simulink model "fbw"  (R2020b)
settings: Solver=FixedStepAuto  StartTime=0.0  StopTime=10.0  FixedStep=0.02  RelTol=1e-3
undefined symbols (not defined in the file): DiscIntNeverNeededParam
libraries: simulink_extras x7, pid_lib x1
settings Model: Creator=Andreas  LastModifiedBy=Andreas

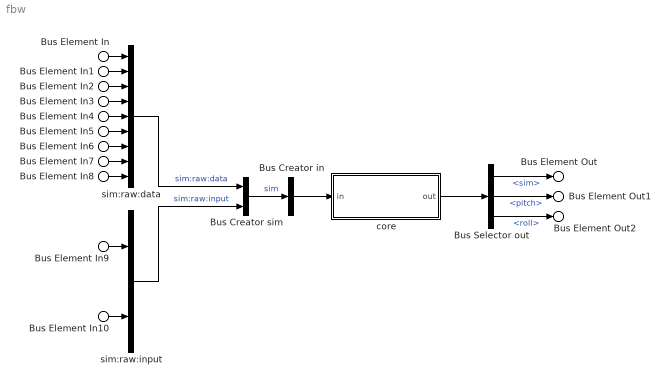
== system fbw ==
  Bus Element In : Inport  PortName=in  Element=sim.sim:raw:data.nz_g
  Bus Element In1 : Inport  PortName=in  Element=sim.sim:raw:data.Theta_deg
  Bus Element In2 : Inport  PortName=in  Element=sim.sim:raw:data.Phi_deg
  Bus Element In3 : Inport  PortName=in  Element=sim.sim:raw:data.qk_rad_s
  Bus Element In4 : Inport  PortName=in  Element=sim.sim:raw:data.rk_rad_s
  Bus Element In5 : Inport  PortName=in  Element=sim.sim:raw:data.pk_rad_s
  Bus Element In6 : Inport  PortName=in  Element=sim.sim:raw:data.Vk_kt
  Bus Element In7 : Inport  PortName=in  Element=sim.sim:raw:data.radio_height_ft
  Bus Element In8 : Inport  PortName=in  Element=sim.sim:raw:data.CG_percent_MAC
  Bus Element In9 : Inport  PortName=in  Element=sim.sim:raw:input.delta_eta_pos
  Bus Element In10 : Inport  PortName=in  Element=sim.sim:raw:input.delta_xi_pos
  Bus Creator sim : BusCreator  Inputs=2
  Bus Creator in : BusCreator  Inputs=1
  Bus Selector out : BusSelector  OutputSignals=sim,pitch,roll
  core : Subsystem
  sim:raw:data : BusCreator  Inputs=9
  sim:raw:input : BusCreator  Inputs=2
  Bus Element Out : Outport  PortName=out  Element=sim
  Bus Element Out1 : Outport  PortName=out  Element=pitch
  Bus Element Out2 : Outport  PortName=out  Element=roll
  wires:
  Bus Element In/1 -> sim:raw:data/1
  sim:raw:data/1 -> Bus Creator sim/1  "sim:raw:data"
  Bus Element In1/1 -> sim:raw:data/2
  Bus Element In2/1 -> sim:raw:data/3
  Bus Element In3/1 -> sim:raw:data/4
  Bus Element In4/1 -> sim:raw:data/5
  Bus Element In5/1 -> sim:raw:data/6
  Bus Element In6/1 -> sim:raw:data/7
  Bus Element In7/1 -> sim:raw:data/8
  Bus Element In8/1 -> sim:raw:data/9
  Bus Element In9/1 -> sim:raw:input/1
  Bus Element In10/1 -> sim:raw:input/2
  sim:raw:input/1 -> Bus Creator sim/2  "sim:raw:input"
  Bus Creator sim/1 -> Bus Creator in/1  "sim"
  Bus Creator in/1 -> core/1(in)
  core/1(out) -> Bus Selector out/1
  Bus Selector out/1 -> Bus Element Out/1  "<sim>"
  Bus Selector out/2 -> Bus Element Out1/1  "<pitch>"
  Bus Selector out/3 -> Bus Element Out2/1  "<roll>"

== system fbw/core ==
  in : Inport
  Data Computation : Subsystem
  Flight Laws : Subsystem
  Normalization : Subsystem
  Reverse Normalization : Subsystem
  out : Outport
  wires:
  Normalization/1(out) -> Data Computation/1(in)
  [B] -> Reverse Normalization/1(in)
  Data Computation/1(out) -> [A]
  [A] -> Flight Laws/1(in)
  Flight Laws/1(out) -> [B]
  Reverse Normalization/1(out) -> out/1
  in/1 -> Normalization/1(in)

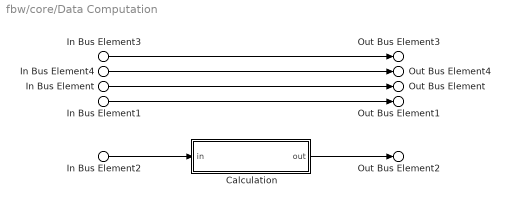
== system fbw/core/Data Computation ==
  In Bus Element2 : Inport  PortName=in
  In Bus Element : Inport  PortName=in  Element=sim.sim:data
  In Bus Element1 : Inport  PortName=in  Element=sim.sim:input
  In Bus Element3 : Inport  PortName=in  Element=sim.sim:raw:data
  In Bus Element4 : Inport  PortName=in  Element=sim.sim:raw:input
  Calculation : Subsystem
  Out Bus Element3 : Outport  PortName=out  Element=sim.sim:raw:data
  Out Bus Element4 : Outport  PortName=out  Element=sim.sim:raw:input
  Out Bus Element : Outport  PortName=out  Element=sim.sim:data
  Out Bus Element2 : Outport  PortName=out  Element=sim.sim:data:computed
  Out Bus Element1 : Outport  PortName=out  Element=sim.sim:input
  wires:
  In Bus Element4/1 -> Out Bus Element4/1
  In Bus Element3/1 -> Out Bus Element3/1
  Calculation/1(out) -> Out Bus Element2/1
  In Bus Element1/1 -> Out Bus Element1/1
  In Bus Element/1 -> Out Bus Element/1
  In Bus Element2/1 -> Calculation/1(in)

== system fbw/core/Flight Laws ==
  In Bus Element3 : Inport  PortName=in
  In Bus Element4 : Inport  PortName=in
  In Bus Element : Inport  PortName=in  Element=sim
  Bus Selector : BusSelector  OutputSignals=roll.roll:data:computed,roll.roll:normal,roll.roll:output  OutputAsBus=on
  Bus Selector1 : BusSelector  OutputSignals=pitch.pitch:data:computed,pitch.pitch:normal,pitch.pitch:protection:attitude:min,pitch.pitch:protection:attitude:max,pitch.pitch:vote,pitch.pitch:integrated,pitch.pitch:output  OutputAsBus=on
  Pitch : Subsystem
  Roll : Subsystem
  Out Bus Element : Outport  PortName=out  Element=sim
  Out Bus Element1 : Outport  PortName=out  Element=pitch
  Out Bus Element2 : Outport  PortName=out  Element=roll
  wires:
  Bus Selector1/1 -> Out Bus Element1/1
  Pitch/1(Output) -> Bus Selector1/1
  Bus Selector/1 -> Out Bus Element2/1
  Roll/1(out) -> Bus Selector/1
  In Bus Element4/1 -> Roll/1(in)
  In Bus Element/1 -> Out Bus Element/1
  In Bus Element3/1 -> Pitch/1(in)

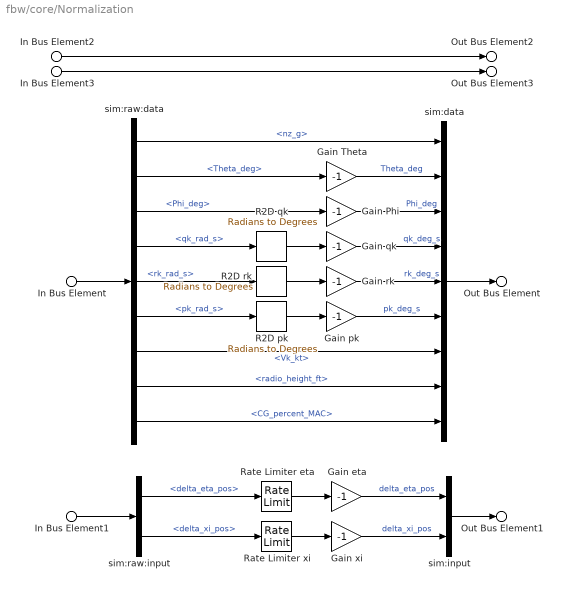
== system fbw/core/Normalization ==
  In Bus Element : Inport  PortName=in  Element=sim.sim:raw:data
  In Bus Element2 : Inport  PortName=in  Element=sim.sim:raw:data
  In Bus Element1 : Inport  PortName=in  Element=sim.sim:raw:input
  In Bus Element3 : Inport  PortName=in  Element=sim.sim:raw:input
  Gain Phi : Gain  Gain=-1
  Gain Theta : Gain  Gain=-1
  Gain eta : Gain  Gain=-1
  Gain pk : Gain  Gain=-1
  Gain qk : Gain  Gain=-1
  Gain rk : Gain  Gain=-1
  Gain xi : Gain  Gain=-1
  R2D pk : simulink_extras/Transformations/Radians to Degrees
  R2D qk : simulink_extras/Transformations/Radians to Degrees
  R2D rk : simulink_extras/Transformations/Radians to Degrees
  Rate Limiter eta : RateLimiter  RisingSlewLimit=10  FallingSlewLimit=-10  SampleTimeMode=inherited
  Rate Limiter xi : RateLimiter  RisingSlewLimit=10  FallingSlewLimit=-10  SampleTimeMode=inherited
  sim:data : BusCreator  Inputs=9
  sim:input : BusCreator  Inputs=2
  sim:raw:data : BusSelector  OutputSignals=nz_g,Theta_deg,Phi_deg,qk_rad_s,rk_rad_s,pk_rad_s,Vk_kt,radio_height_ft,CG_percent_MAC
  sim:raw:input : BusSelector  OutputSignals=delta_eta_pos,delta_xi_pos
  Out Bus Element2 : Outport  PortName=out  Element=sim.sim:raw:data
  Out Bus Element3 : Outport  PortName=out  Element=sim.sim:raw:input
  Out Bus Element : Outport  PortName=out  Element=sim.sim:data
  Out Bus Element1 : Outport  PortName=out  Element=sim.sim:input
  wires:
  In Bus Element3/1 -> Out Bus Element3/1
  In Bus Element2/1 -> Out Bus Element2/1
  Rate Limiter xi/1 -> Gain xi/1
  Rate Limiter eta/1 -> Gain eta/1
  Gain xi/1 -> sim:input/2  "delta_xi_pos"
  Gain eta/1 -> sim:input/1  "delta_eta_pos"
  R2D pk/1 -> Gain pk/1
  R2D rk/1 -> Gain rk/1
  R2D qk/1 -> Gain qk/1
  Gain pk/1 -> sim:data/6  "pk_deg_s"
  Gain rk/1 -> sim:data/5  "rk_deg_s"
  Gain qk/1 -> sim:data/4  "qk_deg_s"
  Gain Phi/1 -> sim:data/3  "Phi_deg"
  Gain Theta/1 -> sim:data/2  "Theta_deg"
  sim:input/1 -> Out Bus Element1/1
  sim:data/1 -> Out Bus Element/1
  sim:raw:input/2 -> Rate Limiter xi/1  "<delta_xi_pos>"
  sim:raw:input/1 -> Rate Limiter eta/1  "<delta_eta_pos>"
  sim:raw:data/9 -> sim:data/9  "<CG_percent_MAC>"
  sim:raw:data/8 -> sim:data/8  "<radio_height_ft>"
  sim:raw:data/7 -> sim:data/7  "<Vk_kt>"
  sim:raw:data/6 -> R2D pk/1  "<pk_rad_s>"
  sim:raw:data/5 -> R2D rk/1  "<rk_rad_s>"
  sim:raw:data/4 -> R2D qk/1  "<qk_rad_s>"
  sim:raw:data/3 -> Gain Phi/1  "<Phi_deg>"
  sim:raw:data/2 -> Gain Theta/1  "<Theta_deg>"
  sim:raw:data/1 -> sim:data/1  "<nz_g>"
  In Bus Element1/1 -> sim:raw:input/1
  In Bus Element/1 -> sim:raw:data/1

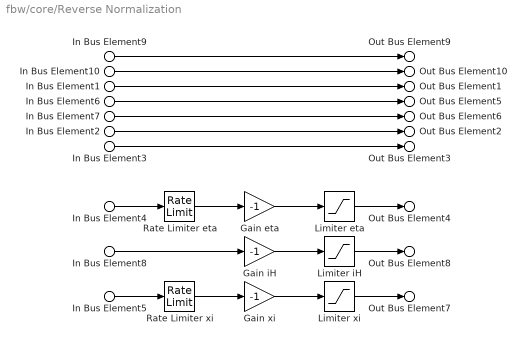
== system fbw/core/Reverse Normalization ==
  In Bus Element1 : Inport  PortName=in  Element=sim.sim:data
  In Bus Element6 : Inport  PortName=in  Element=sim.sim:data:computed
  In Bus Element7 : Inport  PortName=in  Element=sim.sim:input
  In Bus Element9 : Inport  PortName=in  Element=sim.sim:raw:data
  In Bus Element10 : Inport  PortName=in  Element=sim.sim:raw:input
  In Bus Element2 : Inport  PortName=in  Element=pitch
  In Bus Element4 : Inport  PortName=in  Element=pitch.pitch:output.eta_pos
  In Bus Element8 : Inport  PortName=in  Element=pitch.pitch:output.iH_deg
  In Bus Element3 : Inport  PortName=in  Element=roll
  In Bus Element5 : Inport  PortName=in  Element=roll.roll:output.xi_pos
  Gain eta : Gain  Gain=-1
  Gain iH : Gain  Gain=-1
  Gain xi : Gain  Gain=-1
  Limiter eta : Saturate  UpperLimit=1.0  LowerLimit=-1.0
  Limiter iH : Saturate  UpperLimit=13  LowerLimit=-3.5
  Limiter xi : Saturate  UpperLimit=1.0  LowerLimit=-1.0
  Rate Limiter eta : RateLimiter  RisingSlewLimit=2.0  FallingSlewLimit=-2.0  SampleTimeMode=inherited
  Rate Limiter xi : RateLimiter  RisingSlewLimit=2  FallingSlewLimit=-2  SampleTimeMode=inherited
  Out Bus Element9 : Outport  PortName=out  Element=sim.sim:raw:data
  Out Bus Element10 : Outport  PortName=out  Element=sim.sim:raw:input
  Out Bus Element1 : Outport  PortName=out  Element=sim.sim:data
  Out Bus Element5 : Outport  PortName=out  Element=sim.sim:data:computed
  Out Bus Element6 : Outport  PortName=out  Element=sim.sim:input
  Out Bus Element4 : Outport  PortName=out  Element=sim.sim:raw:output.eta_pos
  Out Bus Element8 : Outport  PortName=out  Element=sim.sim:raw:output.iH_deg
  Out Bus Element7 : Outport  PortName=out  Element=sim.sim:raw:output.xi_pos
  Out Bus Element2 : Outport  PortName=out  Element=pitch
  Out Bus Element3 : Outport  PortName=out  Element=roll
  wires:
  In Bus Element10/1 -> Out Bus Element10/1
  In Bus Element9/1 -> Out Bus Element9/1
  In Bus Element8/1 -> Gain iH/1
  Gain iH/1 -> Limiter iH/1
  Limiter iH/1 -> Out Bus Element8/1
  Limiter xi/1 -> Out Bus Element7/1
  Gain xi/1 -> Limiter xi/1
  Gain eta/1 -> Limiter eta/1
  Limiter eta/1 -> Out Bus Element4/1
  Rate Limiter xi/1 -> Gain xi/1
  Rate Limiter eta/1 -> Gain eta/1
  In Bus Element7/1 -> Out Bus Element6/1
  In Bus Element6/1 -> Out Bus Element5/1
  In Bus Element5/1 -> Rate Limiter xi/1
  In Bus Element4/1 -> Rate Limiter eta/1
  In Bus Element3/1 -> Out Bus Element3/1
  In Bus Element1/1 -> Out Bus Element1/1
  In Bus Element2/1 -> Out Bus Element2/1

== system fbw/core/Data Computation/Calculation ==
  In Bus Element : Inport  PortName=in  Element=sim.sim:data.radio_height_ft
  Chart : Stateflow chart  TreatAsAtomicUnit=on
  Out Bus Element : Outport  PortName=out  Element=on_ground
  wires:
  Chart/1(onGround) -> Out Bus Element/1
  In Bus Element/1 -> Chart/1(RadioAltitude)

== system fbw/core/Flight Laws/Pitch ==
  in : Inport
  Automatic Trim : Subsystem
  pitch : Subsystem
  pitch:computed : Subsystem
  pitch:integrated : Subsystem
  pitch:output : Subsystem
  pitch:vote : Subsystem
  Output : Outport
  wires:
  Automatic Trim/1(out) -> Output/1
  [A] -> Automatic Trim/1(in)
  pitch:output/1(out) -> [A]
  pitch:integrated/1(out) -> pitch:output/1(in)
  pitch:vote/1(out) -> pitch:integrated/1(in)
  pitch/1(out) -> pitch:vote/1(in)
  in/1 -> pitch:computed/1(in)
  pitch:computed/1(out) -> pitch/1(in)

== system fbw/core/Flight Laws/Roll ==
  in : Inport
  roll:computed : Subsystem
  roll:normal : Subsystem
  roll:output : Subsystem
  out : Outport
  wires:
  roll:output/1(out) -> out/1
  roll:normal/1(out) -> roll:output/1(in)
  roll:computed/1(out) -> roll:normal/1(in)
  in/1 -> roll:computed/1(in)

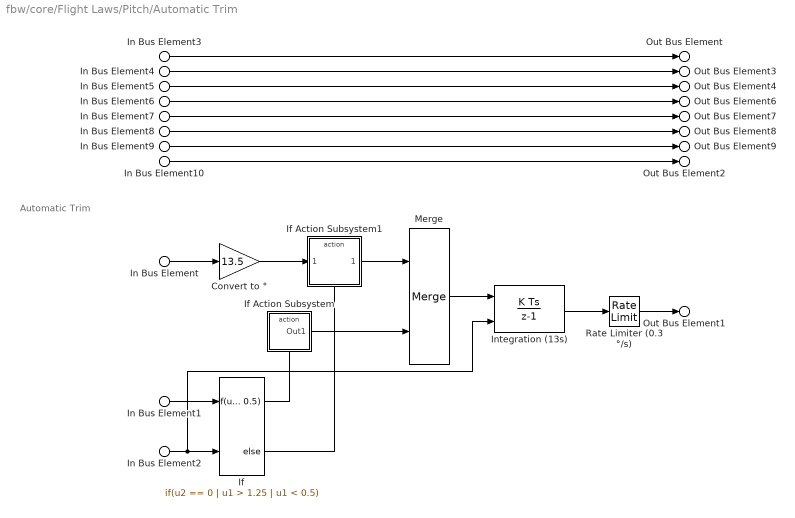
== system fbw/core/Flight Laws/Pitch/Automatic Trim ==
  note: Automatic Trim
  In Bus Element : Inport  PortName=in  Element=pitch.pitch:output.eta_pos
  In Bus Element10 : Inport  PortName=in  Element=pitch.pitch:output.eta_pos
  In Bus Element4 : Inport  PortName=in  Element=pitch.pitch:data:computed
  In Bus Element2 : Inport  PortName=in  Element=pitch.pitch:data:computed.in_flight
  In Bus Element8 : Inport  PortName=in  Element=pitch.pitch:vote
  In Bus Element9 : Inport  PortName=in  Element=pitch.pitch:integrated
  In Bus Element6 : Inport  PortName=in  Element=pitch.pitch:protection:attitude:min
  In Bus Element7 : Inport  PortName=in  Element=pitch.pitch:protection:attitude:max
  In Bus Element5 : Inport  PortName=in  Element=pitch.pitch:normal
  In Bus Element3 : Inport  PortName=in  Element=sim
  In Bus Element1 : Inport  PortName=in  Element=sim.sim:data.nz_g
  Convert to ° : Gain  Gain=13.5
  If : If  NumInputs=2  IfExpression=u2 == 0 | u1 > 1.25 | u1 < 0.5
  If Action Subsystem : Subsystem  TreatAsAtomicUnit=on
  If Action Subsystem1 : Subsystem  TreatAsAtomicUnit=on
  Integration (13s) : DiscreteIntegrator  gainval=1/13  ExternalReset=falling  SampleTime=-1  LimitOutput=on  UpperSaturationLimit=3.5  LowerSaturationLimit=-11  ICPrevOutput=DiscIntNeverNeededParam  ICPrevScaledInput=DiscIntNeverNeededParam
  Merge : Merge
  Rate Limiter (0.3 °/s) : RateLimiter  RisingSlewLimit=0.3  FallingSlewLimit=-0.3  SampleTimeMode=inherited
  Out Bus Element : Outport  PortName=out  Element=sim
  Out Bus Element3 : Outport  PortName=out  Element=pitch.pitch:data:computed
  Out Bus Element4 : Outport  PortName=out  Element=pitch.pitch:normal
  Out Bus Element6 : Outport  PortName=out  Element=pitch.pitch:protection:attitude:min
  Out Bus Element7 : Outport  PortName=out  Element=pitch.pitch:protection:attitude:max
  Out Bus Element8 : Outport  PortName=out  Element=pitch.pitch:vote
  Out Bus Element9 : Outport  PortName=out  Element=pitch.pitch:integrated
  Out Bus Element2 : Outport  PortName=out  Element=pitch.pitch:output.eta_pos
  Out Bus Element1 : Outport  PortName=out  Element=pitch.pitch:output.iH_deg
  wires:
  In Bus Element10/1 -> Out Bus Element2/1
  In Bus Element3/1 -> Out Bus Element/1
  In Bus Element4/1 -> Out Bus Element3/1
  In Bus Element5/1 -> Out Bus Element4/1
  In Bus Element7/1 -> Out Bus Element7/1
  In Bus Element6/1 -> Out Bus Element6/1
  In Bus Element9/1 -> Out Bus Element9/1
  In Bus Element8/1 -> Out Bus Element8/1
  In Bus Element/1 -> Convert to °/1
  If Action Subsystem/1(Out1) -> Merge/2
  In Bus Element1/1 -> If/1
  Integration (13s)/1 -> Rate Limiter (0.3 °/s)/1
  If Action Subsystem1/1(Out1) -> Merge/1
  Merge/1 -> Integration (13s)/1
  If/1 -> If Action Subsystem/Action
  If/2 -> If Action Subsystem1/Action
  In Bus Element2/1 -> Integration (13s)/2, If/2
  Convert to °/1 -> If Action Subsystem1/1(η (°))
  Rate Limiter (0.3 °/s)/1 -> Out Bus Element1/1

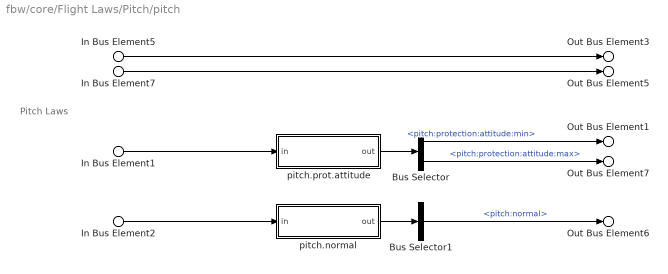
== system fbw/core/Flight Laws/Pitch/pitch ==
  note: Pitch Laws
  In Bus Element1 : Inport  PortName=in
  In Bus Element2 : Inport  PortName=in
  In Bus Element5 : Inport  PortName=in  Element=sim
  In Bus Element7 : Inport  PortName=in  Element=pitch.pitch:data:computed
  Bus Selector : BusSelector  OutputSignals=pitch.pitch:protection:attitude:min,pitch.pitch:protection:attitude:max
  Bus Selector1 : BusSelector  OutputSignals=pitch.pitch:normal
  pitch.normal : Subsystem
  pitch.prot.attitude : Subsystem
  Out Bus Element3 : Outport  PortName=out  Element=sim
  Out Bus Element5 : Outport  PortName=out  Element=pitch.pitch:data:computed
  Out Bus Element6 : Outport  PortName=out  Element=pitch.pitch:normal
  Out Bus Element1 : Outport  PortName=out  Element=pitch.pitch:protection:attitude:min
  Out Bus Element7 : Outport  PortName=out  Element=pitch.pitch:protection:attitude:max
  wires:
  Bus Selector1/1 -> Out Bus Element6/1  "<pitch:normal>"
  Bus Selector/2 -> Out Bus Element7/1  "<pitch:protection:attitude:max>"
  Bus Selector/1 -> Out Bus Element1/1  "<pitch:protection:attitude:min>"
  pitch.normal/1(out) -> Bus Selector1/1
  In Bus Element2/1 -> pitch.normal/1(in)
  pitch.prot.attitude/1(out) -> Bus Selector/1
  In Bus Element1/1 -> pitch.prot.attitude/1(in)
  In Bus Element7/1 -> Out Bus Element5/1
  In Bus Element5/1 -> Out Bus Element3/1

== system fbw/core/Flight Laws/Pitch/pitch:computed ==
  In Bus Element3 : Inport  PortName=in
  In Bus Element1 : Inport  PortName=in  Element=sim
  computation : Subsystem
  Out Bus Element1 : Outport  PortName=out  Element=sim
  Out Bus Element3 : Outport  PortName=out  Element=pitch.pitch:data:computed
  wires:
  computation/1(out) -> Out Bus Element3/1
  In Bus Element3/1 -> computation/1(in)
  In Bus Element1/1 -> Out Bus Element1/1

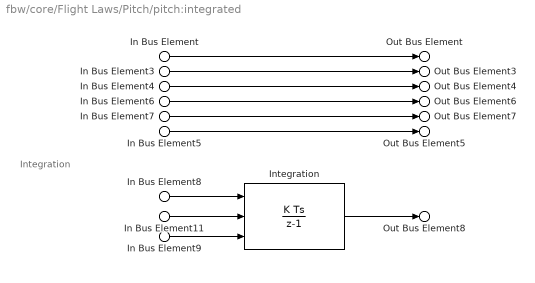
== system fbw/core/Flight Laws/Pitch/pitch:integrated ==
  note: Integration
  In Bus Element : Inport  PortName=in  Element=sim
  In Bus Element9 : Inport  PortName=in  Element=sim.sim:input.delta_eta_pos
  In Bus Element3 : Inport  PortName=in  Element=pitch.pitch:data:computed
  In Bus Element11 : Inport  PortName=in  Element=pitch.pitch:data:computed.in_flight
  In Bus Element6 : Inport  PortName=in  Element=pitch.pitch:protection:attitude:min
  In Bus Element7 : Inport  PortName=in  Element=pitch.pitch:protection:attitude:max
  In Bus Element5 : Inport  PortName=in  Element=pitch.pitch:vote
  In Bus Element8 : Inport  PortName=in  Element=pitch.pitch:vote.eta_dot_pos_s
  In Bus Element4 : Inport  PortName=in  Element=pitch.pitch:normal
  Integration : DiscreteIntegrator  ExternalReset=rising  InitialConditionSource=external  SampleTime=-1  LimitOutput=on  UpperSaturationLimit=1.0  LowerSaturationLimit=-1.0  ICPrevOutput=DiscIntNeverNeededParam  ICPrevScaledInput=DiscIntNeverNeededParam
  Out Bus Element : Outport  PortName=out  Element=sim
  Out Bus Element3 : Outport  PortName=out  Element=pitch.pitch:data:computed
  Out Bus Element4 : Outport  PortName=out  Element=pitch.pitch:normal
  Out Bus Element6 : Outport  PortName=out  Element=pitch.pitch:protection:attitude:min
  Out Bus Element7 : Outport  PortName=out  Element=pitch.pitch:protection:attitude:max
  Out Bus Element5 : Outport  PortName=out  Element=pitch.pitch:vote
  Out Bus Element8 : Outport  PortName=out  Element=pitch.pitch:integrated.eta_pos
  wires:
  In Bus Element9/1 -> Integration/3
  In Bus Element8/1 -> Integration/1
  Integration/1 -> Out Bus Element8/1
  In Bus Element11/1 -> Integration/2
  In Bus Element5/1 -> Out Bus Element5/1
  In Bus Element/1 -> Out Bus Element/1
  In Bus Element3/1 -> Out Bus Element3/1
  In Bus Element4/1 -> Out Bus Element4/1
  In Bus Element7/1 -> Out Bus Element7/1
  In Bus Element6/1 -> Out Bus Element6/1

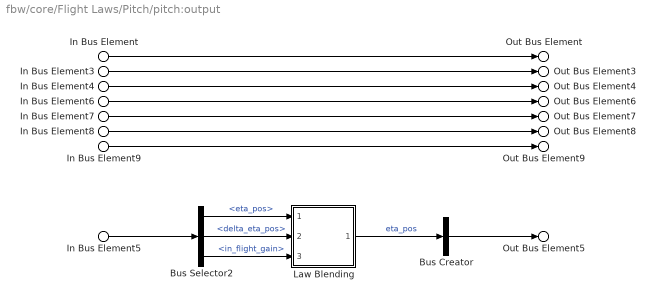
== system fbw/core/Flight Laws/Pitch/pitch:output ==
  In Bus Element5 : Inport  PortName=in
  In Bus Element : Inport  PortName=in  Element=sim
  In Bus Element3 : Inport  PortName=in  Element=pitch.pitch:data:computed
  In Bus Element8 : Inport  PortName=in  Element=pitch.pitch:vote
  In Bus Element9 : Inport  PortName=in  Element=pitch.pitch:integrated
  In Bus Element6 : Inport  PortName=in  Element=pitch.pitch:protection:attitude:min
  In Bus Element7 : Inport  PortName=in  Element=pitch.pitch:protection:attitude:max
  In Bus Element4 : Inport  PortName=in  Element=pitch.pitch:normal
  Bus Creator : BusCreator  Inputs=1
  Bus Selector2 : BusSelector  OutputSignals=pitch.pitch:integrated.eta_pos,sim.sim:input.delta_eta_pos,pitch.pitch:data:computed.in_flight_gain
  Law Blending : Subsystem  ReferencedSubsystem=fbw_law_blending
  Out Bus Element : Outport  PortName=out  Element=sim
  Out Bus Element3 : Outport  PortName=out  Element=pitch.pitch:data:computed
  Out Bus Element4 : Outport  PortName=out  Element=pitch.pitch:normal
  Out Bus Element6 : Outport  PortName=out  Element=pitch.pitch:protection:attitude:min
  Out Bus Element7 : Outport  PortName=out  Element=pitch.pitch:protection:attitude:max
  Out Bus Element8 : Outport  PortName=out  Element=pitch.pitch:vote
  Out Bus Element9 : Outport  PortName=out  Element=pitch.pitch:integrated
  Out Bus Element5 : Outport  PortName=out  Element=pitch.pitch:output
  wires:
  In Bus Element9/1 -> Out Bus Element9/1
  In Bus Element8/1 -> Out Bus Element8/1
  In Bus Element7/1 -> Out Bus Element7/1
  In Bus Element6/1 -> Out Bus Element6/1
  Bus Creator/1 -> Out Bus Element5/1
  Law Blending/1 -> Bus Creator/1  "eta_pos"
  In Bus Element5/1 -> Bus Selector2/1
  Bus Selector2/3 -> Law Blending/3  "<in_flight_gain>"
  Bus Selector2/2 -> Law Blending/2  "<delta_eta_pos>"
  Bus Selector2/1 -> Law Blending/1  "<eta_pos>"
  In Bus Element4/1 -> Out Bus Element4/1
  In Bus Element3/1 -> Out Bus Element3/1
  In Bus Element/1 -> Out Bus Element/1

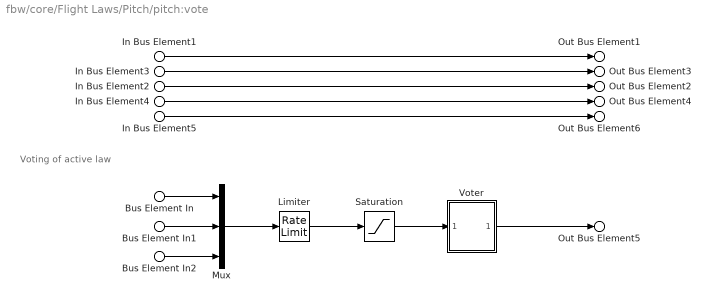
== system fbw/core/Flight Laws/Pitch/pitch:vote ==
  note: Voting of active law
  In Bus Element1 : Inport  PortName=in  Element=sim
  In Bus Element3 : Inport  PortName=in  Element=pitch.pitch:data:computed
  In Bus Element2 : Inport  PortName=in  Element=pitch.pitch:normal
  Bus Element In : Inport  PortName=in  Element=pitch.pitch:normal.eta_dot_pos_s
  In Bus Element4 : Inport  PortName=in  Element=pitch.pitch:protection:attitude:min
  Bus Element In1 : Inport  PortName=in  Element=pitch.pitch:protection:attitude:min.eta_dot_pos_s
  In Bus Element5 : Inport  PortName=in  Element=pitch.pitch:protection:attitude:max
  Bus Element In2 : Inport  PortName=in  Element=pitch.pitch:protection:attitude:max.eta_dot_pos_s
  Limiter : RateLimiter  RisingSlewLimit=30  FallingSlewLimit=-30  SampleTimeMode=inherited
  Mux : Mux  Inputs=3
  Saturation : Saturate  UpperLimit=5  LowerLimit=-5
  Voter : MATLAB Function  TreatAsAtomicUnit=on
  Out Bus Element1 : Outport  PortName=out  Element=sim
  Out Bus Element3 : Outport  PortName=out  Element=pitch.pitch:data:computed
  Out Bus Element2 : Outport  PortName=out  Element=pitch.pitch:normal
  Out Bus Element4 : Outport  PortName=out  Element=pitch.pitch:protection:attitude:min
  Out Bus Element6 : Outport  PortName=out  Element=pitch.pitch:protection:attitude:max
  Out Bus Element5 : Outport  PortName=out  Element=pitch.pitch:vote.eta_dot_pos_s
  wires:
  In Bus Element5/1 -> Out Bus Element6/1
  In Bus Element4/1 -> Out Bus Element4/1
  In Bus Element2/1 -> Out Bus Element2/1
  Voter/1(vote) -> Out Bus Element5/1
  Saturation/1 -> Voter/1(input)
  Limiter/1 -> Saturation/1
  Bus Element In2/1 -> Mux/3
  Bus Element In/1 -> Mux/1
  Mux/1 -> Limiter/1
  Bus Element In1/1 -> Mux/2
  In Bus Element3/1 -> Out Bus Element3/1
  In Bus Element1/1 -> Out Bus Element1/1

== system fbw/core/Flight Laws/Roll/roll:computed ==
  In Bus Element3 : Inport  PortName=in
  In Bus Element1 : Inport  PortName=in  Element=sim
  computation : Subsystem
  Out Bus Element1 : Outport  PortName=out  Element=sim
  Out Bus Element3 : Outport  PortName=out  Element=roll.roll:data:computed
  wires:
  computation/1(out) -> Out Bus Element3/1
  In Bus Element3/1 -> computation/1(in)
  In Bus Element1/1 -> Out Bus Element1/1

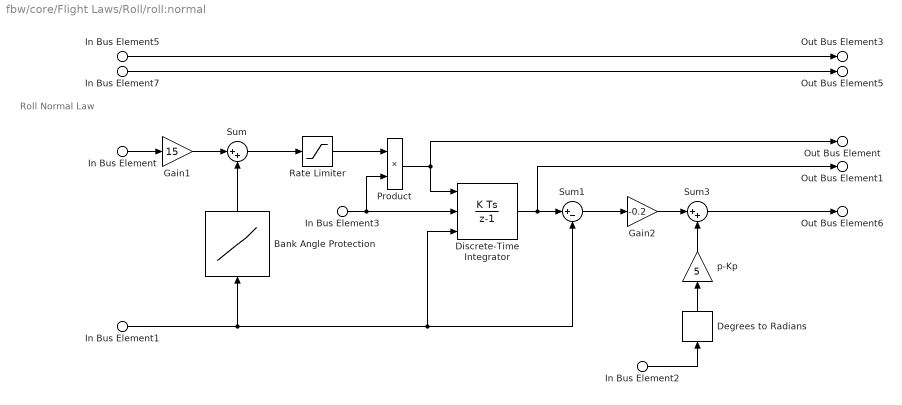
== system fbw/core/Flight Laws/Roll/roll:normal ==
  note: Roll Normal Law
  In Bus Element5 : Inport  PortName=in  Element=sim
  In Bus Element : Inport  PortName=in  Element=sim.sim:input.delta_xi_pos
  In Bus Element1 : Inport  PortName=in  Element=sim.sim:data.Phi_deg
  In Bus Element2 : Inport  PortName=in  Element=sim.sim:data.pk_deg_s
  In Bus Element7 : Inport  PortName=in  Element=roll.roll:data:computed
  In Bus Element3 : Inport  PortName=in  Element=roll.roll:data:computed.in_flight
  Bank Angle Protection : Lookup_n-D  NumberOfTableDimensions=1  BreakpointsForDimension1=[-90,-66,-33,0,33,66,90]  Table=[15,15,0,0,0,-15,-15]  InternalRulePriority=Speed  RndMeth=Simplest  InputSameDT=on
  Degrees to Radians : simulink_extras/Transformations/Degrees to Radians
  Discrete-Time Integrator : DiscreteIntegrator  ExternalReset=rising  InitialConditionSource=external  SampleTime=-1  LimitOutput=on  UpperSaturationLimit=66  LowerSaturationLimit=-66  ICPrevOutput=DiscIntNeverNeededParam  ICPrevScaledInput=DiscIntNeverNeededParam
  Gain1 : Gain  Gain=15
  Gain2 : Gain  Gain=-0.2
  Product : Product
  Rate Limiter : Saturate  UpperLimit=15  LowerLimit=-15
  Sum : Sum  Inputs=|++
  Sum1 : Sum  Inputs=|+-
  Sum3 : Sum  Inputs=|++
  p-Kp : Gain  Gain=5
  Out Bus Element3 : Outport  PortName=out  Element=sim
  Out Bus Element5 : Outport  PortName=out  Element=roll.roll:data:computed
  Out Bus Element : Outport  PortName=out  Element=roll.roll:normal.pk_c_deg_s
  Out Bus Element1 : Outport  PortName=out  Element=roll.roll:normal.Phi_c_deg
  Out Bus Element6 : Outport  PortName=out  Element=roll.roll:normal.xi_pos
  wires:
  In Bus Element7/1 -> Out Bus Element5/1
  In Bus Element5/1 -> Out Bus Element3/1
  In Bus Element2/1 -> Degrees to Radians/1
  In Bus Element1/1 -> Bank Angle Protection/1, Discrete-Time Integrator/3, Sum1/2
  In Bus Element/1 -> Gain1/1
  Product/1 -> Discrete-Time Integrator/1, Out Bus Element/1
  Rate Limiter/1 -> Product/1
  In Bus Element3/1 -> Discrete-Time Integrator/2, Product/2
  Discrete-Time Integrator/1 -> Sum1/1, Out Bus Element1/1
  Degrees to Radians/1 -> p-Kp/1
  Sum3/1 -> Out Bus Element6/1
  Gain1/1 -> Sum/1
  Sum1/1 -> Gain2/1
  Gain2/1 -> Sum3/1
  p-Kp/1 -> Sum3/2
  Bank Angle Protection/1 -> Sum/2
  Sum/1 -> Rate Limiter/1

== system fbw/core/Flight Laws/Roll/roll:output ==
  In Bus Element5 : Inport  PortName=in
  In Bus Element1 : Inport  PortName=in  Element=sim
  In Bus Element3 : Inport  PortName=in  Element=roll.roll:data:computed
  In Bus Element4 : Inport  PortName=in  Element=roll.roll:normal
  Bus Selector2 : BusSelector  OutputSignals=roll.roll:normal.xi_pos,sim.sim:input.delta_xi_pos,roll.roll:data:computed.in_flight_gain
  Law Blending : Subsystem  ReferencedSubsystem=fbw_law_blending
  Out Bus Element1 : Outport  PortName=out  Element=sim
  Out Bus Element3 : Outport  PortName=out  Element=roll.roll:data:computed
  Out Bus Element4 : Outport  PortName=out  Element=roll.roll:normal
  Out Bus Element : Outport  PortName=out  Element=roll.roll:output.xi_pos
  wires:
  Law Blending/1 -> Out Bus Element/1
  In Bus Element5/1 -> Bus Selector2/1
  Bus Selector2/3 -> Law Blending/3  "<in_flight_gain>"
  Bus Selector2/2 -> Law Blending/2  "<delta_xi_pos>"
  Bus Selector2/1 -> Law Blending/1  "<xi_pos>"
  In Bus Element4/1 -> Out Bus Element4/1
  In Bus Element3/1 -> Out Bus Element3/1
  In Bus Element1/1 -> Out Bus Element1/1

== system fbw/core/Flight Laws/Pitch/Automatic Trim/If Action Subsystem ==
  Action Port : ActionPort  InitializeStates=reset
  Constant : Constant  Value=0
  Out1 : Outport
  wires:
  Constant/1 -> Out1/1

== system fbw/core/Flight Laws/Pitch/Automatic Trim/If Action Subsystem1 ==
  η (°) : Inport
  Action Port : ActionPort
  Out1 : Outport
  wires:
  η (°)/1 -> Out1/1

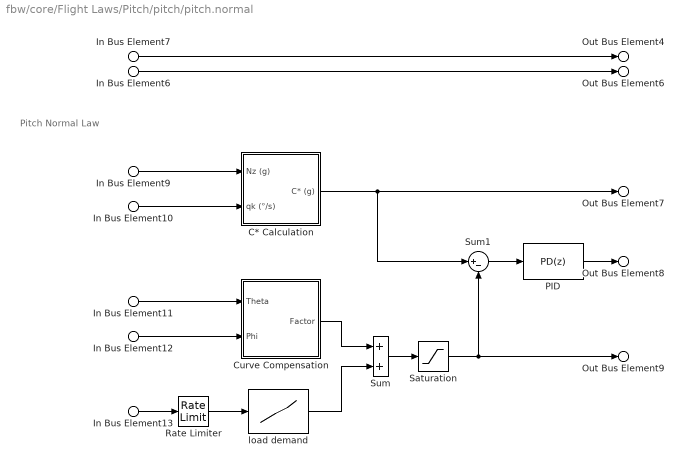
== system fbw/core/Flight Laws/Pitch/pitch/pitch.normal ==
  note: Pitch Normal Law
  In Bus Element7 : Inport  PortName=in  Element=sim
  In Bus Element13 : Inport  PortName=in  Element=sim.sim:input.delta_eta_pos
  In Bus Element12 : Inport  PortName=in  Element=sim.sim:data.Phi_deg
  In Bus Element11 : Inport  PortName=in  Element=sim.sim:data.Theta_deg
  In Bus Element10 : Inport  PortName=in  Element=sim.sim:data.qk_deg_s
  In Bus Element9 : Inport  PortName=in  Element=sim.sim:data.nz_g
  In Bus Element6 : Inport  PortName=in  Element=pitch.pitch:data:computed
  C* Calculation : Subsystem
      mask Display:
      | disp('')
      | port_label('input', 1, 'N_z [g]','interpreter','tex')
      | port_label('input', 2, 'q [°/s]','interpreter','tex')
      | port_label('output', 1, 'C* [g]','interpreter','tex')
  Curve Compensation : Subsystem
      mask Display:
      | disp('')
      | port_label('input', 1, '\Theta [°]','interpreter','tex')
      | port_label('input', 2, '\Phi [°]','interpreter','tex')
      | port_label('output', 1, 'Factor','interpreter','tex')
  PID : pid_lib/PID Controller  Controller=PD  Form=Parallel  TimeDomain=Discrete-time  UseExternalTs=off  SampleTime=-1  IntegratorMethod=Forward Euler  FilterMethod=Forward Euler  ControllerParametersSource=internal  P=0.450  I=0  D=0.200  UseFilter=off  N=100  TunerSelectOption=Transfer Function Based (PID Tuner App)  InitialConditionSource=internal  InitialConditionForIntegrator=0  InitialConditionForFilter=0  DifferentiatorICPrevScaledInput=0  ExternalReset=none  TrackingMode=off  Kt=1  LimitOutput=on  SatLimitsSource=internal  UpperSaturationLimit=1.0  LowerSaturationLimit=-1.0  LinearizeAsGain=off  AntiWindupMode=clamping  Kb=1  POutMin=[]  POutMax=[]  IOutMin=[]  IOutMax=[]  DOutMin=[]  DOutMax=[]  NOutMin=[]  NOutMax=[]  SumOutMin=[]  SumOutMax=[]  SaturationOutMin=[]  SaturationOutMax=[]  PParamMin=[]  PParamMax=[]  IParamMin=[]  IParamMax=[]  DParamMin=[]  DParamMax=[]  NParamMin=[]  NParamMax=[]  KbParamMin=[]  KbParamMax=[]  KtParamMin=[]  KtParamMax=[]  KbOutMin=[]  KbOutMax=[]  KtOutMin=[]  KtOutMax=[]  IntegratorOutMin=[]  IntegratorOutMax=[]  FilterOutMin=[]  FilterOutMax=[]  SumI1OutMin=[]  SumI1OutMax=[]  SumI2OutMin=[]  SumI2OutMax=[]  SumI3OutMin=[]  SumI3OutMax=[]  SumI4OutMin=[]  SumI4OutMax=[]  SumDOutMin=[]  SumDOutMax=[]  DifferentiatorOutMin=[]  DifferentiatorOutMax=[]  FilterDiffOutCoefMin=[]  FilterDiffOutCoefMax=[]  ReciprocalOutMin=[]  ReciprocalOutMax=[]  SumDenOutMin=[]  SumDenOutMax=[]  SumNumOutMin=[]  SumNumOutMax=[]  DivideOutMin=[]  DivideOutMax=[]  UdiffTsProdOutMin=[]  UdiffTsProdOutMax=[]  NTsProdOutMin=[]  NTsProdOutMax=[]  UintegralTsProdOutMin=[]  UintegralTsProdOutMax=[]  UngainTsProdOutMin=[]  UngainTsProdOutMax=[]  IntegratorContinuousStateAttributes=''  IntegratorStateMustResolveToSignalObject=off  IntegratorRTWStateStorageClass=Auto  FilterContinuousStateAttributes=''  FilterStateMustResolveToSignalObject=off  FilterRTWStateStorageClass=Auto  ParallelPVariant=InternalParameters  IdealPVariant=Disabled  IVariant=Disabled  DVariant=InternalParameters  IntegratorVariant=Disabled  SatVariant=Enabled  AWVariant=Disabled  PCopyVariant=Disabled  TRVariant=Disabled  FdbkBlocksVariant=Forward  IdealPFdbkVariant=Disabled  SatFdbkVariant=Disabled  DerivativeFilterVariant=Differentiator  NVariant=Passthrough  NCopyVariant=Disabled_SignalSpec  FilterICVariant=InternalICsDifferentiator  IntegratorICVariant=Disabled  ExternalResetVariant=Disabled  TRSumVariant=Passthrough  SumFdbkVariant=Disabled  SumVariant=Sum_PD  TsampFilterVariant=InternalTs  TsampNgainVariant=Passthrough  TsampIntegralVariant=Disabled_SignalSpec  ExternalSaturationOutDataTypeStr=Inherit: Same as second input
  Rate Limiter : RateLimiter  RisingSlewLimit=0.75  FallingSlewLimit=-0.75  SampleTimeMode=inherited
  Saturation : Saturate  UpperLimit=2.5  LowerLimit=-1.0
  Sum : Sum
  Sum1 : Sum  Inputs=|+-
  load demand : Lookup_n-D  NumberOfTableDimensions=1  BreakpointsForDimension1=[-1 0 1]  Table=[-2 0 1.5]  InternalRulePriority=Speed  RndMeth=Simplest  InputSameDT=on
  Out Bus Element4 : Outport  PortName=out  Element=sim
  Out Bus Element6 : Outport  PortName=out  Element=pitch.pitch:data:computed
  Out Bus Element7 : Outport  PortName=out  Element=pitch.pitch:normal.Cstar_g
  Out Bus Element9 : Outport  PortName=out  Element=pitch.pitch:normal.Cstar_c_g
  Out Bus Element8 : Outport  PortName=out  Element=pitch.pitch:normal.eta_dot_pos_s
  wires:
  In Bus Element7/1 -> Out Bus Element4/1
  In Bus Element6/1 -> Out Bus Element6/1
  In Bus Element13/1 -> Rate Limiter/1
  In Bus Element12/1 -> Curve Compensation/2(Phi)
  In Bus Element9/1 -> C* Calculation/1(Nz (g))
  Saturation/1 -> Sum1/2, Out Bus Element9/1
  Rate Limiter/1 -> load demand/1
  In Bus Element10/1 -> C* Calculation/2(qk (°/s))
  PID/1 -> Out Bus Element8/1
  In Bus Element11/1 -> Curve Compensation/1(Theta)
  Sum/1 -> Saturation/1
  load demand/1 -> Sum/2
  C* Calculation/1(C* (g)) -> Sum1/1, Out Bus Element7/1
  Curve Compensation/1(Factor) -> Sum/1
  Sum1/1 -> PID/1

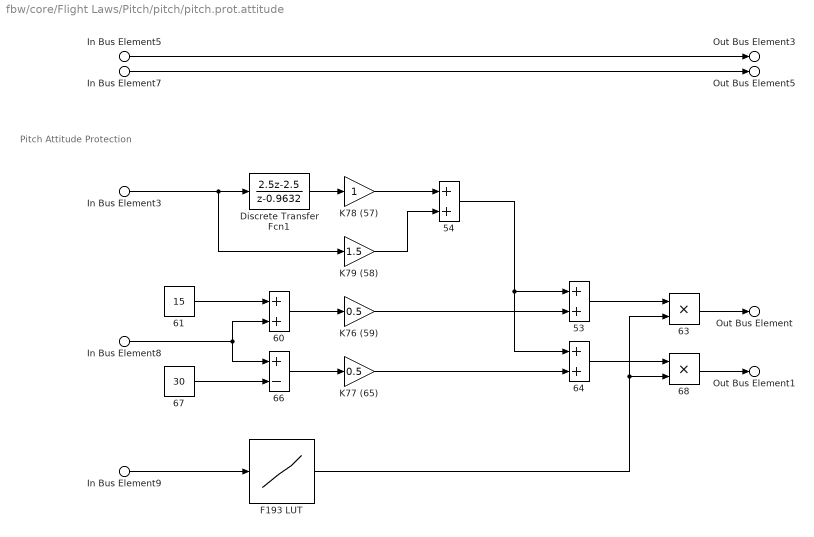
== system fbw/core/Flight Laws/Pitch/pitch/pitch.prot.attitude ==
  note: Pitch Attitude Protection
  In Bus Element5 : Inport  PortName=in  Element=sim
  In Bus Element3 : Inport  PortName=in  Element=sim.sim:data.qk_deg_s
  In Bus Element8 : Inport  PortName=in  Element=sim.sim:data.Theta_deg
  In Bus Element9 : Inport  PortName=in  Element=sim.sim:data.Vk_kt
  In Bus Element7 : Inport  PortName=in  Element=pitch.pitch:data:computed
  {53..54,60,64} (4 alike) : Sum
  61 : Constant  Value=15
  63 : Product
  66 : Sum  Inputs=+-
  67 : Constant  Value=30
  68 : Product
  Discrete Transfer Fcn1 : DiscreteTransferFcn  Numerator=[2.5 -2.5]  Denominator=[1 -0.9632]
  F193 LUT : Lookup_n-D  NumberOfTableDimensions=1  BreakpointsForDimension1=[0 120 130 160 190 210 280 350]  Table=[2.2 2.2 1.9 1.35 1.05 0.58 0.45 0.41]  InternalRulePriority=Speed  RndMeth=Simplest  InputSameDT=on
  K76 (59) : Gain  Gain=0.5
  K77 (65) : Gain  Gain=0.5
  K78 (57) : Gain
  K79 (58) : Gain  Gain=1.5
  Out Bus Element3 : Outport  PortName=out  Element=sim
  Out Bus Element5 : Outport  PortName=out  Element=pitch.pitch:data:computed
  Out Bus Element : Outport  PortName=out  Element=pitch.pitch:protection:attitude:min.eta_dot_pos_s
  Out Bus Element1 : Outport  PortName=out  Element=pitch.pitch:protection:attitude:max.eta_dot_pos_s
  wires:
  In Bus Element7/1 -> Out Bus Element5/1
  In Bus Element5/1 -> Out Bus Element3/1
  In Bus Element8/1 -> 66/1, 60/2
  F193 LUT/1 -> 63/2, 68/2
  In Bus Element9/1 -> F193 LUT/1
  63/1 -> Out Bus Element/1
  68/1 -> Out Bus Element1/1
  64/1 -> 68/1
  53/1 -> 63/1
  54/1 -> 53/1, 64/1
  K76 (59)/1 -> 53/2
  K77 (65)/1 -> 64/2
  67/1 -> 66/2
  61/1 -> 60/1
  66/1 -> K77 (65)/1
  60/1 -> K76 (59)/1
  Discrete Transfer Fcn1/1 -> K78 (57)/1
  In Bus Element3/1 -> K79 (58)/1, Discrete Transfer Fcn1/1
  K79 (58)/1 -> 54/2
  K78 (57)/1 -> 54/1

== system fbw/core/Flight Laws/Pitch/pitch:computed/computation ==
  In Bus Element : Inport  PortName=in  Element=sim.sim:data.Theta_deg
  In Bus Element2 : Inport  PortName=in  Element=sim.sim:data.radio_height_ft
  In Bus Element1 : Inport  PortName=in  Element=sim.sim:data:computed.on_ground
  Chart1 : Stateflow chart  TreatAsAtomicUnit=on
  Rate Limit : RateLimiter  RisingSlewLimit=1/5  FallingSlewLimit=-1/5  SampleTimeMode=inherited
  Saturation : Saturate  UpperLimit=1  LowerLimit=0
  Out Bus Element : Outport  PortName=out  Element=in_flight
  Out Bus Element1 : Outport  PortName=out  Element=in_flare
  Out Bus Element2 : Outport  PortName=out  Element=in_flight_gain
  wires:
  Rate Limit/1 -> Out Bus Element2/1
  Chart1/1(inFlight) -> Out Bus Element/1, Saturation/1
  Saturation/1 -> Rate Limit/1
  In Bus Element1/1 -> Chart1/3(on_ground)
  In Bus Element2/1 -> Chart1/2(radio_height)
  In Bus Element/1 -> Chart1/1(Theta)
  Chart1/2(inFlare) -> Out Bus Element1/1

== system fbw/core/Flight Laws/Roll/roll:computed/computation ==
  In Bus Element : Inport  PortName=in  Element=sim.sim:data.Theta_deg
  In Bus Element2 : Inport  PortName=in  Element=sim.sim:data.radio_height_ft
  In Bus Element1 : Inport  PortName=in  Element=sim.sim:data:computed.on_ground
  Chart : Stateflow chart  TreatAsAtomicUnit=on
  Rate Limit : RateLimiter  RisingSlewLimit=1/0.5  FallingSlewLimit=-1/0.5  SampleTimeMode=inherited
  Saturation : Saturate  UpperLimit=1  LowerLimit=0
  Out Bus Element : Outport  PortName=out  Element=in_flight
  Out Bus Element2 : Outport  PortName=out  Element=in_flight_gain
  wires:
  Saturation/1 -> Rate Limit/1
  Rate Limit/1 -> Out Bus Element2/1
  Chart/1(inFlight) -> Out Bus Element/1, Saturation/1
  In Bus Element/1 -> Chart/1(Theta)
  In Bus Element1/1 -> Chart/2(on_ground)
  In Bus Element2/1 -> Chart/3(radio_height)

== system fbw/core/Flight Laws/Pitch/pitch/pitch.normal/C* Calculation ==
  Nz (g) : Inport
  qk (°/s) : Inport  Port=2
  Constant2 : Constant  Value=121/9.81
  Degrees to Radians : simulink_extras/Transformations/Degrees to Radians
  Product : Product
  Sum : Sum  Inputs=|++
  C* (g) : Outport
  wires:
  Constant2/1 -> Product/2
  Degrees to Radians/1 -> Product/1
  Product/1 -> Sum/2
  qk (°/s)/1 -> Degrees to Radians/1
  Nz (g)/1 -> Sum/1
  Sum/1 -> C* (g)/1

== system fbw/core/Flight Laws/Pitch/pitch/pitch.normal/Curve Compensation ==
  Theta : Inport
  Phi : Inport  Port=2
  Cos : Trigonometry  Operator=cos
  Cos1 : Trigonometry  Operator=cos
  Degrees to Radians : simulink_extras/Transformations/Degrees to Radians
  Degrees to Radians1 : simulink_extras/Transformations/Degrees to Radians
  Divide : Product  Inputs=*/
  Factor : Outport
  wires:
  Degrees to Radians1/1 -> Cos1/1
  Degrees to Radians/1 -> Cos/1
  Divide/1 -> Factor/1
  Cos1/1 -> Divide/2
  Cos/1 -> Divide/1
  Phi/1 -> Degrees to Radians1/1
  Theta/1 -> Degrees to Radians/1

== stateflow chart fbw/core/Data Computation/Calculation/Chart ==
  state OnGround
    onGround = 1;
  state InAir
    onGround = 0;
  OnGround -> InAir : [RadioAltitude > 10]
  (default) -> OnGround
  InAir -> OnGround : [RadioAltitude <= 10]
  data: RadioAltitude input; onGround output

== stateflow chart fbw/core/Flight Laws/Pitch/pitch:computed/computation/Chart1 ==
  state Ground
    inFlight = 0;
    inFlare = 0;
  state Flight_Low
    inFlight = 1;
    inFlare = 0;
  state Flight_High
    inFlight = 1;
    inFlare = 0;
  state Flare
    inFlight = 1;
    inFlare = 1;
  Flight_Low -> Flight_High : [radio_height > 50]
  Ground -> Flight_Low : [(on_ground == 0 & Theta > 8) | radio_height > 400]
  (default) -> Ground
  Flare -> Ground [order 1] : [duration(on_ground == 1 & Theta < 2.5) > 5]
  Flare -> Flight_Low [order 2] : [radio_height > 50 & Theta > 8]
  Flight_High -> Flare : [radio_height <= 50]
  data: Theta input; radio_height input; inFlight output; inFlare output; on_ground input

== matlab function fbw/core/Flight Laws/Pitch/pitch:vote/Voter ==
  data: input input; vote output
function vote = Voter(input)
vote = median(input);

== stateflow chart fbw/core/Flight Laws/Roll/roll:computed/computation/Chart ==
  state GroundMode
    inFlight = 0;
  state FlightMode
    inFlight = 1;
  GroundMode -> FlightMode : [(on_ground == 0 & Theta > 8) | radio_height > 400]
  (default) -> GroundMode
  FlightMode -> GroundMode : [on_ground == 1]
  data: Theta input; on_ground input; inFlight output; radio_height input
